simulink model "mppt_fuzzy"  (R2023b)
settings: Solver=VariableStepAuto  StartTime=0.0  StopTime=0.2  RelTol=1e-3
libraries: spsSeriesRLCBranchLib x3, spsDiodeLib x2, fuzblock x1, spsPWMGeneratorDCDCLib x1, spsMosfetLib x1, spsPVArrayLib x1, spsSeriesRLCLoadLib x1, spsVoltageMeasurementLib x1, spspowerguiLib x1
settings Model: SimulationMode=accelerator  Creator=KUNA JASWANTHINI  LastModifiedBy=chand
settings OptimizationCC: ReuseModelBlockBuffer=off
settings DebuggingCC: UnconnectedInputMsg=warning  UnconnectedOutputMsg=warning  UnconnectedLineMsg=warning
settings ModelReferenceCC: EnableRefExpFcnMdlSchedulingChecks=on
settings RTWCC: DLArmComputeVersion=19.05

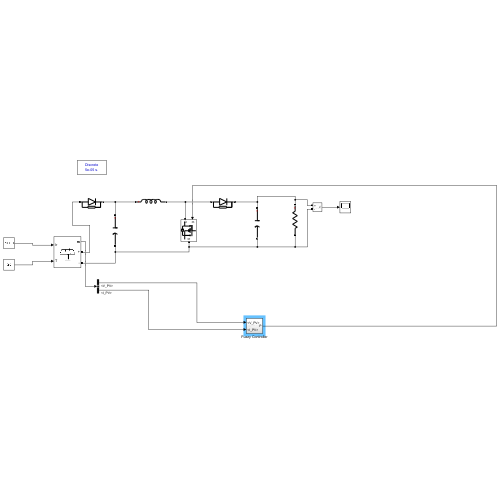
[thumbnail: Simulink's stored preview of the top-level diagram]
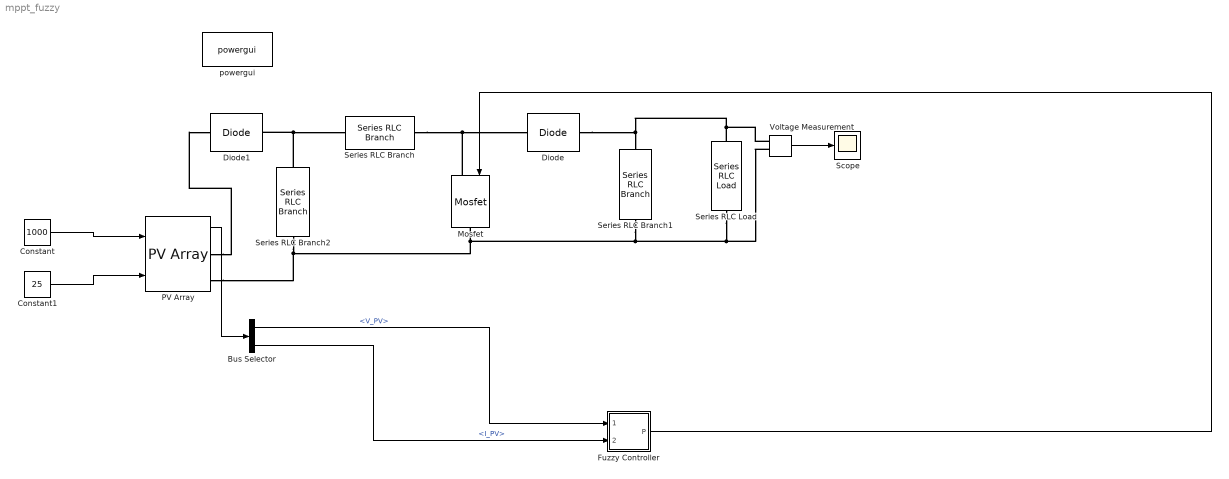
== system mppt_fuzzy ==
  Bus Selector : BusSelector  OutputSignals=V_PV,I_PV
  Constant : Constant  Value=1000
  Constant1 : Constant  Value=25
  Diode : spsDiodeLib/Diode  Ron=0.001  Lon=0  Vf=0.8  IC=0  UseSnubber=0  Rs=500  Cs=250e-9  Measurements=off
  Diode1 : spsDiodeLib/Diode  Ron=0.001  Lon=0  Vf=0.8  IC=0  UseSnubber=0  Rs=500  Cs=250e-9  Measurements=off
  Fuzzy Controller : Subsystem
  Mosfet : spsMosfetLib/Mosfet  Ron=0.1  Lon=0  Rd=0.01  Vfd=0  IC=0  Rs=1e5  Cs=inf  Measurements=off
  PV Array : spsPVArrayLib/PV Array  Npar=4  Nser=2  PlotType=one module @ 25 deg.C & specified irradiances  S_vec=[1000 800 500 250]  Temp_C_vec="[ 1000 800 500 250   ]"  ModuleName=Waaree Energies WU-120  PlotWhenSelected=off  Pm=120.7  Ncell=72  Voc=21  Isc=8  Vm=17  Im=7.1  beta_Voc_pc=-0.358  alpha_Isc_pc=0.052  beta_Voc=-0.07518  alpha_Isc=0.00416  IL=8.0502  I0=2.411e-10  nI=0.47063  Rsh=31.6819  Rs=0.19891  RobustModel=off  RobustCellTemperature=313.3991  BAL=on  Tc=1e-6  Tfilter=5e-5
  Scope : Scope
  Series RLC Branch : spsSeriesRLCBranchLib/Series RLC Branch  LConnTagsString=__new0  RConnTagsString=__new0  BranchType=L  Resistance=1  Inductance=1e-4  SetiL0=off  InitialCurrent=0  Capacitance=1e-6  Setx0=off  InitialVoltage=0  Measurements=None
  Series RLC Branch1 : spsSeriesRLCBranchLib/Series RLC Branch  LConnTagsString=__new0  RConnTagsString=__new0  BranchType=C  Resistance=1  Inductance=1e-4  SetiL0=off  InitialCurrent=0  Capacitance=50e-6  Setx0=off  InitialVoltage=0  Measurements=None
  Series RLC Branch2 : spsSeriesRLCBranchLib/Series RLC Branch  LConnTagsString=__new0  RConnTagsString=__new0  BranchType=C  Resistance=1  Inductance=1e-4  SetiL0=off  InitialCurrent=0  Capacitance=4000e-6  Setx0=off  InitialVoltage=0  Measurements=None
  Series RLC Load : spsSeriesRLCLoadLib/Series RLC Load  LConnTagsString=a  RConnTagsString=__new0  NominalVoltage=30  NominalFrequency=50  ActivePower=120  InductivePower=0  CapacitivePower=0  Setx0=off  InitialVoltage=0  SetiL0=off  InitialCurrent=0  Measurements=None  LoadType=constant Z
  Voltage Measurement : spsVoltageMeasurementLib/Voltage Measurement  PhasorSimulation=off  OutputType=Complex  PSBequivalent=0
  powergui : spspowerguiLib/powergui  Priority=1  SimulationMode=Discrete  SampleTime=50e-6  frequency=60  Iterations=50  frequencyindice=0  Pbase=100e6  ErrMax=1e-4  UnitsV=kV  UnitsW=MW  buscounter=0  FunctionMessages=off  echomessages=off  EnableUseOfTLC=off  CurrentSourceSwitches=off  DisableSnubberDevices=off  DisableRonSwitches=off  DisableVfSwitches=off  DisplayEquations=off  AutomaticDiscreteSolvers=off  SolverType=Tustin/Backward Euler (TBE)  Interpol=off  ExternalGateDelay=off  methode=off  Ts=100  x0status=blocks  SPID=on  SwTol=0  HookPort=off  NonlinearTolerance=1e-4  nMaxIteration=100  ContinueOnMaxIteration=off  RestoreLinks=warning  ResistiveCurrentMeasurement=off  Frange=[0:2:500]  Ylog=off  Xlog=on  ShowGrid=off  save=off  variable=ZData  structure=0  ZoomFFT=off  StartTime=0.0  cycles=1  DisplayStyle=1  fundamental=60  FreqAxis=off  MaxFrequency=1000  frequencyindicesteady=1  RmsSteady=1  display=off
  wires:
  Constant/1 -> PV Array/1
  Constant1/1 -> PV Array/2
  PV Array/1 -> Bus Selector/1
  Voltage Measurement/1 -> Scope/1
  Bus Selector/1 -> Fuzzy Controller/1(<V_PV>)  "<V_PV>"
  Bus Selector/2 -> Fuzzy Controller/2(<I_PV>)  "<I_PV>"
  Fuzzy Controller/1(P) -> Mosfet/1
  connections:
  Series RLC Branch2/LConn1 -- Series RLC Branch/LConn1 -- Diode1/RConn1
  Series RLC Branch/RConn1 -- Mosfet/LConn1 -- Diode/LConn1
  Series RLC Branch2/RConn1 -- PV Array/RConn2 -- Series RLC Load/RConn1 -- Voltage Measurement/LConn2 -- Series RLC Branch1/RConn1 -- Mosfet/RConn1
  Diode/RConn1 -- Voltage Measurement/LConn1 -- Series RLC Load/LConn1 -- Series RLC Branch1/LConn1
  PV Array/RConn1 -- Diode1/LConn1

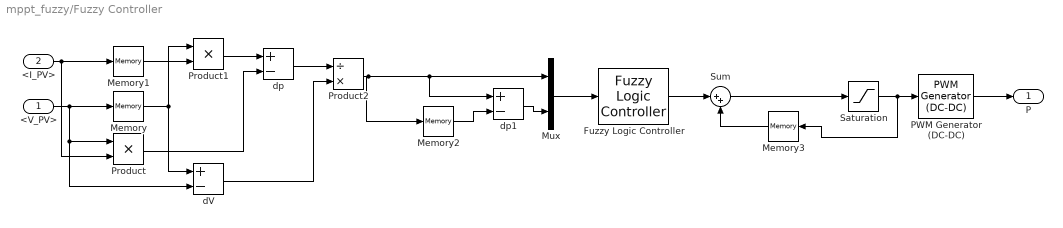
== system mppt_fuzzy/Fuzzy Controller ==
  <V_PV> : Inport
  <I_PV> : Inport  Port=2
  Fuzzy Logic Controller : fuzblock/Fuzzy Logic  Controller  FIS="\"C:\\Users\\ugopa\\OneDrive\\Desktop\\Raji Project\\mppt using fuzzy\\mppt_fuzzy.fis\""  OutputSampleNumber=101  DataType=double  FuzzifiedInputs=off  RuleFiringStrengths=off  RuleOutputs=off  AggregatedOutputs=off  SimulateUsing=Interpreted execution  OutOfRangeInputValueMessage=warning  NoRuleFiredMessage=warning  EmptyOutputFuzzySetMessage=warning
  Memory{,1..3} (4 alike) : Memory
  Mux : Mux  Inputs=2
  PWM Generator (DC-DC) : spsPWMGeneratorDCDCLib/PWM Generator (DC-DC)  Fsw=5000  Ts=0
  Product : Product
  Product1 : Product
  Product2 : Product  Inputs=/*
  Saturation : Saturate
  Sum : Sum  Inputs=|++
  dV : Sum  Inputs=+-
  dp : Sum  Inputs=+-
  dp1 : Sum  Inputs=+-
  P : Outport
  wires:
  <I_PV>/1 -> Memory1/1, Product/2
  dp/1 -> Product2/1
  dV/1 -> Product2/2
  <V_PV>/1 -> dV/2, Product/1, Memory/1
  Product/1 -> dp/2
  Memory1/1 -> Product1/2
  Memory/1 -> dV/1, Product1/1
  Mux/1 -> Fuzzy Logic Controller/1
  Product1/1 -> dp/1
  Sum/1 -> Saturation/1
  Product2/1 -> Mux/1, dp1/1, Memory2/1
  Memory2/1 -> dp1/2
  Memory3/1 -> Sum/2
  dp1/1 -> Mux/2
  Fuzzy Logic Controller/1 -> Sum/1
  Saturation/1 -> Memory3/1, PWM Generator (DC-DC)/1
  PWM Generator (DC-DC)/1 -> P/1
